simulink model "MVC2026_sim"  (R2023b)
settings: Solver=ode23t  StartTime=0.0  StopTime=inf  FixedStep=Ts  RelTol=1e-3
values from neighbouring files (symbols this model uses):
  saveDataSampling = 0.01    [main.m]
undefined symbols (not defined in the file or in its folder): BAT, BUS, CH, CTRLpmsm, DiscIntNeverNeededParam, EMS, LoadRef, MOT, TraceRef, Ts, VEH, WindRef
libraries: nesl_utility x50, fl_lib x28, ee_lib x19, simulink x9, slpidlib x5, eeTransforms x4, sdl_lib x4, batteryecm_lib x1, eeGeneralControl x1
(part 3 of 3)

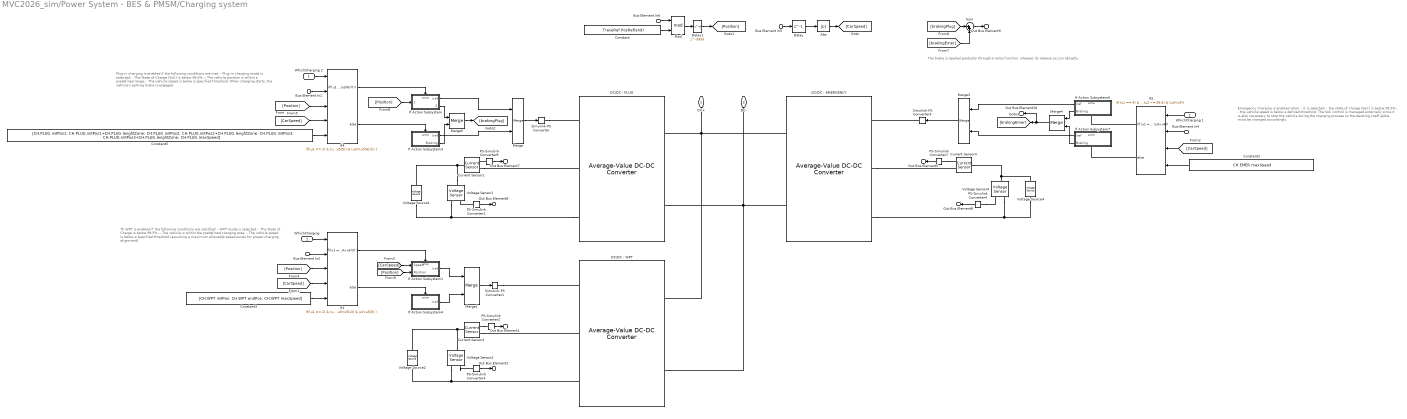
== system MVC2026_sim/Power System - BES & PMSM/Charging system ==
  note: Plug-in charging is enabled if the following conditions are met:
      | - Plug-in charging mode is selected;
      | - The State of Charge (SoC) is below 99.5%;
      | - The vehicle position is within a predefined range;
      | - The vehicle speed is below a specified threshold.
      |
      | When charging starts, the vehicle’s parking brake is engaged.
  note: Th WPT is enabled if the following conditions are satisfied:
      | - WPT mode is selected;
      | - The State of Charge is below 99.5%;
      | - The vehicle is within the predefined charging area;
      | - The vehicle speed is below a specified threshold (assuming a maximum
      |  allowable speed exists for proper charging alignment).
  note: Emergency charging is enabled when:
      | - it is selected;
      | - the state of charge (SoC) is below 99.5%;
      | - the vehicle speed is below a defined threshold.
      |
      | The SoC control is managed externally since it is also necessary
      | to stop the vehicle during the charging process so the derating coeff alpha
      | must be changed accordingly.
  note: The brake is applied gradually through a ramp function, whereas its release occurs abruptly.
  WhichCharging : Inport
  Bus Element In4 : Inport  Port=2  PortName=DAQ  Element=SoC_BP
  Bus Element In1 : Inport  Port=2  PortName=DAQ  Element=SoC_BP
  Bus Element In2 : Inport  Port=2  PortName=DAQ  Element=SoC_BP
  Bus Element In6 : Inport  Port=2  PortName=DAQ  Element=Position
  Bus Element In5 : Inport  Port=2  PortName=DAQ  Element=CarSpeed
  Abs : Abs  SaturateOnIntegerOverflow=off
  Constant : Constant  Value=TraceRef.PosRef(end)
  Constant2 : Constant  Value=CH.EMER.maxSpeed
  Constant3 : Constant  Value=[CH.WPT.initPos; CH.WPT.endPos; CH.WPT.maxSpeed]
  Constant5 : Constant  Value=[CH.PLUG.initPos1; CH.PLUG.initPos1+CH.PLUG.lenghtZone; CH.PLUG.initPos2; CH.PLUG.initPos2+CH.PLUG.lenghtZone; CH.PLUG.initPos3; CH.PLUG.initPos3+CH.PLUG.lenghtZone; CH.PLUG.maxSpeed]
  Current Sensor1 : fl_lib/Electrical/Electrical Sensors/Current Sensor
  Current Sensor2 : fl_lib/Electrical/Electrical Sensors/Current Sensor
  Current Sensor4 : fl_lib/Electrical/Electrical Sensors/Current Sensor
  DC/DC - EMERGENCY : ee_lib/Semiconductors & Converters/Converters/Average-Value DC-DC Converter  control_option=ee.enum.converters.controlinput.current  converter_type=ee.enum.converters.dcdctype.buck  efficiency_option=ee.enum.converters.efficiency.tabulated  efficiency_fixed=100  i_vec=CONV.EMER.I A  efficiency_vec=CONV.EMER.eta
      settings: InternalSimscapePortConfiguration="{\"Bottom\":[],\"Left\":[{\"id\":\"Iref\",\"label\":\"Iref\",\"type\":\"input\"},{\"id\":\"p1\",\"label\":\"1+\",\"type\":\"foundation.electrical.electrical\"},{\"id\":\"n1\",\"label\":\"1-\",\"type\":\"foundation.electrical.electrical\"}],\"Right\":[{\"id\":\"p2\",\"label\":\"2+\",\"type\":\"foundation.electrical.electrical\"},{\"id\":\"n2\",\"label\":\"2-\",\"type\":\"foundation.electrical.electrical\"}],\"Top\":[]}"
  DC/DC - PLUG : ee_lib/Semiconductors & Converters/Converters/Average-Value DC-DC Converter  control_option=ee.enum.converters.controlinput.current  converter_type=ee.enum.converters.dcdctype.buck  efficiency_option=ee.enum.converters.efficiency.tabulated  efficiency_fixed=100  i_vec=CONV.PLUG.I A  efficiency_vec=CONV.PLUG.eta
      settings: InternalSimscapePortConfiguration="{\"Bottom\":[],\"Left\":[{\"id\":\"Iref\",\"label\":\"Iref\",\"type\":\"input\"},{\"id\":\"p1\",\"label\":\"1+\",\"type\":\"foundation.electrical.electrical\"},{\"id\":\"n1\",\"label\":\"1-\",\"type\":\"foundation.electrical.electrical\"}],\"Right\":[{\"id\":\"p2\",\"label\":\"2+\",\"type\":\"foundation.electrical.electrical\"},{\"id\":\"n2\",\"label\":\"2-\",\"type\":\"foundation.electrical.electrical\"}],\"Top\":[]}"
  DC/DC - WPT : ee_lib/Semiconductors & Converters/Converters/Average-Value DC-DC Converter  control_option=ee.enum.converters.controlinput.current  converter_type=ee.enum.converters.dcdctype.buck  efficiency_option=ee.enum.converters.efficiency.tabulated  efficiency_fixed=100  i_vec=CONV.WPT.I A  efficiency_vec=CONV.WPT.eta
      settings: InternalSimscapePortConfiguration="{\"Bottom\":[],\"Left\":[{\"id\":\"Iref\",\"label\":\"Iref\",\"type\":\"input\"},{\"id\":\"p1\",\"label\":\"1+\",\"type\":\"foundation.electrical.electrical\"},{\"id\":\"n1\",\"label\":\"1-\",\"type\":\"foundation.electrical.electrical\"}],\"Right\":[{\"id\":\"p2\",\"label\":\"2+\",\"type\":\"foundation.electrical.electrical\"},{\"id\":\"n2\",\"label\":\"2-\",\"type\":\"foundation.electrical.electrical\"}],\"Top\":[]}"
  Delay : Delay  DelayLength=1  SampleTime=Ts
  Delay1 : Delay  DelayLength=3333  UseCircularBuffer=on  SampleTime=Ts
  If Action Subsystem : Subsystem  TreatAsAtomicUnit=on
  If Action Subsystem1 : Subsystem  TreatAsAtomicUnit=on
  If Action Subsystem3 : Subsystem  TreatAsAtomicUnit=on
  If Action Subsystem4 : Subsystem  TreatAsAtomicUnit=on
  If Action Subsystem6 : Subsystem  TreatAsAtomicUnit=on
  If Action Subsystem7 : Subsystem  TreatAsAtomicUnit=on
  If1 : If  NumInputs=5  IfExpression=(u1 == 2) & (u2 <= 99.5) & (u3>u5(1) & u3<u5(2)) & u4<u5(3)
  If3 : If  NumInputs=4  IfExpression=(u1 == 4) & (u2 <= 99.5) & (u3<u4)
  If4 : If  NumInputs=5  IfExpression=(u1 == 1) & (u2 <= 99.5) & (u4<u5(7)) & (((u3>u5(1)) & (u3<(u5(2)))) | ((u3>u5(3)) & (u3<(u5(4)))) | ((u3>u5(5)) & (u3<(u5(6)))))
  Merge{,1,3..5} (5 alike) : Merge
  Mod : Math  Operator=mod
  PS-Simulink Converter1 : nesl_utility/PS-Simulink Converter  PhysicalDomain=network_engine_domain  SubClassName=ps_output  LeftPortType=input  RightPortType=output  PseudoPeriodic=off  Frequencies=[]  VectorFormat=1-D array  Unit=V  AffineConversion=off
  PS-Simulink Converter2 : nesl_utility/PS-Simulink Converter  PhysicalDomain=network_engine_domain  SubClassName=ps_output  LeftPortType=input  RightPortType=output  PseudoPeriodic=off  Frequencies=[]  VectorFormat=1-D array  Unit=A  AffineConversion=off
  PS-Simulink Converter3 : nesl_utility/PS-Simulink Converter  PhysicalDomain=network_engine_domain  SubClassName=ps_output  LeftPortType=input  RightPortType=output  PseudoPeriodic=off  Frequencies=[]  VectorFormat=1-D array  Unit=V  AffineConversion=off
  PS-Simulink Converter4 : nesl_utility/PS-Simulink Converter  PhysicalDomain=network_engine_domain  SubClassName=ps_output  LeftPortType=input  RightPortType=output  PseudoPeriodic=off  Frequencies=[]  VectorFormat=1-D array  Unit=V  AffineConversion=off
  PS-Simulink Converter7 : nesl_utility/PS-Simulink Converter  PhysicalDomain=network_engine_domain  SubClassName=ps_output  LeftPortType=input  RightPortType=output  PseudoPeriodic=off  Frequencies=[]  VectorFormat=1-D array  Unit=A  AffineConversion=off
  PS-Simulink Converter9 : nesl_utility/PS-Simulink Converter  PhysicalDomain=network_engine_domain  SubClassName=ps_output  LeftPortType=input  RightPortType=output  PseudoPeriodic=off  Frequencies=[]  VectorFormat=1-D array  Unit=A  AffineConversion=off
  Simulink-PS Converter : nesl_utility/Simulink-PS Converter  PhysicalDomain=network_engine_domain  SubClassName=ps_input  LeftPortType=input  RightPortType=output  PseudoPeriodic=off  Frequencies=[]  NoiseDistribution=none  NoiseParameters=[]  Unit=A  AffineConversion=off  FilteringAndDerivatives=provide  SimscapeFilterOrder=1  InputFilterTimeConstant=0.001  UdotUserProvided=0
  Simulink-PS Converter1 : nesl_utility/Simulink-PS Converter  PhysicalDomain=network_engine_domain  SubClassName=ps_input  LeftPortType=input  RightPortType=output  PseudoPeriodic=off  Frequencies=[]  NoiseDistribution=none  NoiseParameters=[]  Unit=A  AffineConversion=off  FilteringAndDerivatives=provide  SimscapeFilterOrder=1  InputFilterTimeConstant=0.001  UdotUserProvided=0
  Simulink-PS Converter3 : nesl_utility/Simulink-PS Converter  PhysicalDomain=network_engine_domain  SubClassName=ps_input  LeftPortType=input  RightPortType=output  PseudoPeriodic=off  Frequencies=[]  NoiseDistribution=none  NoiseParameters=[]  Unit=A  AffineConversion=off  FilteringAndDerivatives=provide  SimscapeFilterOrder=1  InputFilterTimeConstant=0.001  UdotUserProvided=0
  Sum : Sum  Inputs=|++
  Voltage Sensor1 : fl_lib/Electrical/Electrical Sensors/Voltage Sensor
  Voltage Sensor2 : fl_lib/Electrical/Electrical Sensors/Voltage Sensor
  Voltage Sensor4 : fl_lib/Electrical/Electrical Sensors/Voltage Sensor
  Voltage Source1 : ee_lib/Sources/Voltage Source  dc_voltage=CH.PLUG.V V  ac_voltage=0 V  ac_shift=0 rad  ac_frequency=60 Hz  noise_mode=ee.enum.sources.noise.Disabled  PSD=0 V^2/Hz  sample_time=1e-3 s  repeatability=ee.enum.sources.repeatability.NotRepeatable  user_seed=0  auto_seed=545404223  i_specify=off  i_priority=None  i=0 A  i_nominal_specify=off  i_nominal_unit=A  i_nominal_value=1  v_specify=off  v_priority=None  v=0 V  v_nominal_specify=off  v_nominal_unit=V  v_nominal_value=1
  Voltage Source2 : ee_lib/Sources/Voltage Source  dc_voltage=CH.WPT.V V  ac_voltage=0 V  ac_shift=0 rad  ac_frequency=60 Hz  noise_mode=ee.enum.sources.noise.Disabled  PSD=0 V^2/Hz  sample_time=1e-3 s  repeatability=ee.enum.sources.repeatability.NotRepeatable  user_seed=0  auto_seed=3922919431  i_specify=off  i_priority=None  i=0 A  i_nominal_specify=off  i_nominal_unit=A  i_nominal_value=1  v_specify=off  v_priority=None  v=0 V  v_nominal_specify=off  v_nominal_unit=V  v_nominal_value=1
  Voltage Source4 : ee_lib/Sources/Voltage Source  dc_voltage=CH.EMER.V V  ac_voltage=0 V  ac_shift=0 rad  ac_frequency=60 Hz  noise_mode=ee.enum.sources.noise.Disabled  PSD=0 V^2/Hz  sample_time=1e-3 s  repeatability=ee.enum.sources.repeatability.NotRepeatable  user_seed=0  auto_seed=4144164703  i_specify=off  i_priority=None  i=0 A  i_nominal_specify=off  i_nominal_unit=A  i_nominal_value=1  v_specify=off  v_priority=None  v=0 V  v_nominal_specify=off  v_nominal_unit=V  v_nominal_value=1
  WhichCharging 1 : InportShadow
  WhichCharging 2 : InportShadow
  DC+ : PMIOPort  Side=Right
  DC- : PMIOPort  Port=2  Side=Right
  Out Bus Element7 : Outport  PortName=CH  Element=iPLUG
  Out Bus Element8 : Outport  PortName=CH  Element=vPLUG
  Out Bus Element1 : Outport  PortName=CH  Element=iWPT
  Out Bus Element2 : Outport  PortName=CH  Element=vWPT
  Out Bus Element5 : Outport  PortName=CH  Element=iEMERGENCY
  Out Bus Element6 : Outport  PortName=CH  Element=vEMERGENCY
  Out Bus Element9 : Outport  PortName=CH  Element=Braking
  Out Bus Element10 : Outport  PortName=CH  Element=EMERGENCYisON
  wires:
  WhichCharging 2/1 -> If4/1
  Bus Element In1/1 -> If4/2
  Bus Element In2/1 -> If1/2
  WhichCharging/1 -> If1/1
  If4/1 -> If Action Subsystem/Action
  If4/2 -> If Action Subsystem3/Action
  If Action Subsystem3/1(Iref) -> Merge/2
  If Action Subsystem/1(Iref) -> Merge/1
  If Action Subsystem1/1(Iref) -> Merge1/1
  If Action Subsystem4/1(Iref) -> Merge1/2
  If1/2 -> If Action Subsystem4/Action
  If1/1 -> If Action Subsystem1/Action
  Merge1/1 -> Simulink-PS Converter1/1
  Bus Element In6/1 -> Mod/1
  Constant/1 -> Mod/2
  Bus Element In5/1 -> Delay/1
  Delay/1 -> Abs/1
  Merge3/1 -> Simulink-PS Converter3/1
  If Action Subsystem/2(Braking) -> Merge5/1
  If Action Subsystem3/2(Braking) -> Merge5/2
  Constant5/1 -> If4/5
  If Action Subsystem7/2(Braking) -> Merge4/2
  If Action Subsystem6/2(Braking) -> Merge4/1
  If3/2 -> If Action Subsystem7/Action
  If Action Subsystem7/1(Iref) -> Merge3/2
  If Action Subsystem6/1(Iref) -> Merge3/1
  If3/1 -> If Action Subsystem6/Action
  Bus Element In4/1 -> If3/2
  Constant2/1 -> If3/4
  Merge4/1 -> Out Bus Element10/1, [brakingEmer]
  Constant3/1 -> If1/5
  Sum/1 -> Out Bus Element9/1
  Abs/1 -> [CarSpeed]
  [CarSpeed] -> If3/3
  [Position] -> If1/3
  [Position] -> If4/3
  Merge5/1 -> [brakingPlug]
  WhichCharging 1/1 -> If3/1
  [Position] -> If Action Subsystem/1(Position)
  [CarSpeed] -> If4/4
  [CarSpeed] -> If1/4
  [CarSpeed] -> If Action Subsystem1/1(Speed)
  Mod/1 -> Delay1/1
  Delay1/1 -> [Position]
  Merge/1 -> Simulink-PS Converter/1
  [brakingEmer] -> Sum/2
  [brakingPlug] -> Sum/1
  [Position] -> If Action Subsystem1/2(Position)
  PS-Simulink Converter9/1 -> Out Bus Element7/1
  PS-Simulink Converter1/1 -> Out Bus Element8/1
  PS-Simulink Converter2/1 -> Out Bus Element1/1
  PS-Simulink Converter3/1 -> Out Bus Element2/1
  PS-Simulink Converter4/1 -> Out Bus Element6/1
  PS-Simulink Converter7/1 -> Out Bus Element5/1
  connections:
  PS-Simulink Converter9/LConn1 -- Current Sensor1/RConn1
  Voltage Sensor1/LConn1 -- Voltage Source1/LConn1 -- Current Sensor1/LConn1
  PS-Simulink Converter1/LConn1 -- Voltage Sensor1/RConn1
  DC/DC - PLUG/LConn3 -- Voltage Source1/RConn1 -- Voltage Sensor1/RConn2
  Current Sensor1/RConn2 -- DC/DC - PLUG/LConn2
  Voltage Source2/LConn1 -- Voltage Sensor2/LConn1 -- Current Sensor2/LConn1
  Current Sensor2/RConn2 -- DC/DC - WPT/LConn2
  Voltage Sensor2/RConn1 -- PS-Simulink Converter3/LConn1
  Current Sensor2/RConn1 -- PS-Simulink Converter2/LConn1
  Voltage Source2/RConn1 -- Voltage Sensor2/RConn2 -- DC/DC - WPT/LConn3
  DC/DC - PLUG/RConn2 -- DC/DC - WPT/RConn2 -- DC/DC - EMERGENCY/RConn2 -- DC-/RConn1
  Simulink-PS Converter/RConn1 -- DC/DC - PLUG/LConn1
  Simulink-PS Converter1/RConn1 -- DC/DC - WPT/LConn1
  Simulink-PS Converter3/RConn1 -- DC/DC - EMERGENCY/LConn1
  Voltage Source4/LConn1 -- Current Sensor4/LConn1 -- Voltage Sensor4/LConn1
  Voltage Source4/RConn1 -- DC/DC - EMERGENCY/LConn3 -- Voltage Sensor4/RConn2
  PS-Simulink Converter4/LConn1 -- Voltage Sensor4/RConn1
  PS-Simulink Converter7/LConn1 -- Current Sensor4/RConn1
  DC/DC - EMERGENCY/LConn2 -- Current Sensor4/RConn2
  DC/DC - WPT/RConn1 -- DC/DC - PLUG/RConn1 -- DC/DC - EMERGENCY/RConn1 -- DC+/RConn1

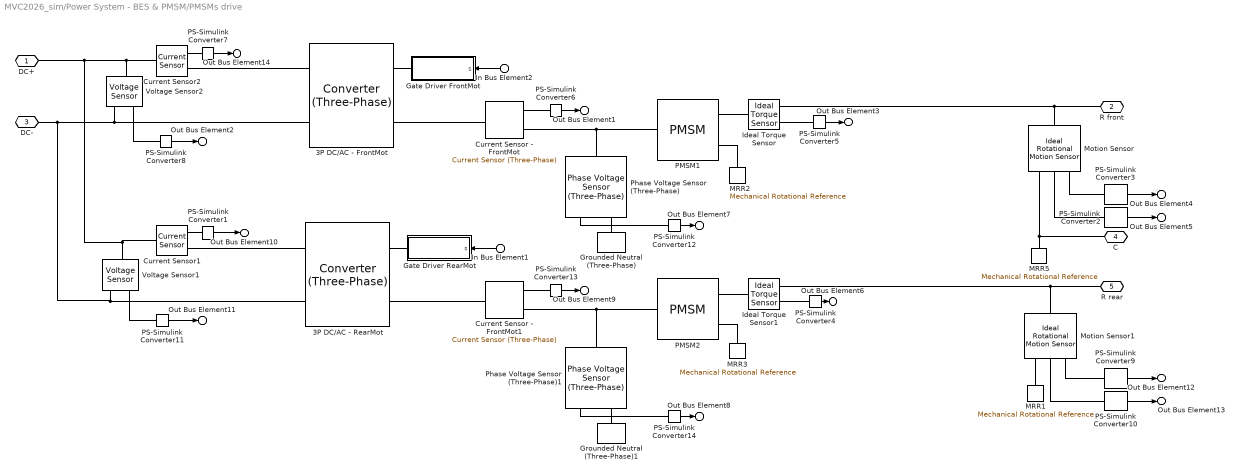
== system MVC2026_sim/Power System - BES & PMSM/PMSMs drive ==
  In Bus Element1 : Inport  PortName=CTRL  Element=swRearMot
  In Bus Element2 : Inport  PortName=CTRL  Element=swFrontMot
  3P DC/AC - FrontMot : ee_lib/Semiconductors & Converters/Converters/Converter (Three-Phase)  port_option=ee.enum.threePhasePort.composite  device_type=ee.enum.converters.switchingdevice.averaged  K=0  Vf=0.01 V  Ron=0.001 Ohm  Rds=0.001 Ohm  Goff=1e-6 1/Ohm  Vgt=1 V  Vgt_off=-1 V  Ih=1 A  Vth=0.5 V  diode_param=ee.enum.converters.protectiondiode.none  diode_Vf=0.8 V  diode_Ron=0.001 Ohm  diode_Goff=1e-5 1/Ohm  diode_C=50 nF  diode_iRM=-235 A  diode_iF=300 A  diode_idot=-50 A/us  diode_trr_param=ee.enum.converters.diodetrr.trr_factor  diode_trr_factor=3  diode_trr=15 us  diode_Qrr=1500 s*uA  snubber_type=ee.enum.converters.snubber.exclude  Cs=1e-7 F  Rs=0.1 Ohm
  3P DC/AC - RearMot : ee_lib/Semiconductors & Converters/Converters/Converter (Three-Phase)  port_option=ee.enum.threePhasePort.composite  device_type=ee.enum.converters.switchingdevice.averaged  K=0  Vf=0.01 V  Ron=0.001 Ohm  Rds=0.001 Ohm  Goff=1e-6 1/Ohm  Vgt=1 V  Vgt_off=-1 V  Ih=1 A  Vth=0.5 V  diode_param=ee.enum.converters.protectiondiode.none  diode_Vf=0.01 V  diode_Ron=0.001 Ohm  diode_Goff=1e-5 1/Ohm  diode_C=50 nF  diode_iRM=-235 A  diode_iF=300 A  diode_idot=-50 A/us  diode_trr_param=ee.enum.converters.diodetrr.trr_factor  diode_trr_factor=3  diode_trr=15 us  diode_Qrr=1500 s*uA  snubber_type=ee.enum.converters.snubber.exclude  Cs=1e-7 F  Rs=0.1 Ohm
  Current Sensor - FrontMot : ee_lib/Sensors & Transducers/Current Sensor (Three-Phase)
  Current Sensor - FrontMot1 : ee_lib/Sensors & Transducers/Current Sensor (Three-Phase)
  Current Sensor1 : fl_lib/Electrical/Electrical Sensors/Current Sensor
  Current Sensor2 : fl_lib/Electrical/Electrical Sensors/Current Sensor
  Gate Driver FrontMot : Subsystem
  Gate Driver RearMot : Subsystem
  Grounded Neutral (Three-Phase) : ee_lib/Connectors & References/Grounded Neutral (Three-Phase)
  Grounded Neutral (Three-Phase)1 : ee_lib/Connectors & References/Grounded Neutral (Three-Phase)
  Ideal Torque Sensor : fl_lib/Mechanical/Mechanical Sensors/Ideal Torque Sensor
  Ideal Torque Sensor1 : fl_lib/Mechanical/Mechanical Sensors/Ideal Torque Sensor
  MRR{1..3,5} (4 alike) : fl_lib/Mechanical/Rotational Elements/Mechanical Rotational Reference
  Motion Sensor : fl_lib/Mechanical/Mechanical Sensors/Ideal Rotational Motion Sensor  reference=foundation.enum.MeasurementReference.difference  acceleration_port=false  velocity_port=true  position_port=true  wrap_angle=simscape.enum.onoff.off  offset=0 rad
  Motion Sensor1 : fl_lib/Mechanical/Mechanical Sensors/Ideal Rotational Motion Sensor  reference=foundation.enum.MeasurementReference.difference  acceleration_port=false  velocity_port=true  position_port=true  wrap_angle=simscape.enum.onoff.off  offset=0 rad
  PMSM1 : ee_lib/Electromechanical/Permanent Magnet/PMSM  port_option=ee.enum.threePhasePort.composite  winding_type=ee.enum.statorconnection.wye  machine_param=ee.enum.pmsm.parameterization.constant  nPolePairs=MOT.Front.p  pmflux_param=ee.enum.pmflux.fluxlinkage  pm_flux_linkage=MOT.Front.PMflux Wb  torque_constant=0.18 N*m/A  back_emf_constant=0.18 V*s/rad  stator_param=ee.enum.statorparam.LdLqL0  Ld=MOT.Front.Ld H  Lq=MOT.Front.Lq H  idVec=[-200, 0, 200] A  iqVec=[-200, 0, 200] A  LdMatrix=0.0002 * ones(3, 3) H  LqMatrix=0.0002 * ones(3, 3) H  PmMatrix=0.1 * ones(3, 3) Wb  ktMatrix=0.18 * ones(3, 3) N*m/A  keMatrix=0.18 * ones(3, 3) V*s/rad  L0=MOT.L0 H  Ls=0.0002 H  Lm=-0.00002 H  Ms=0.00002 H  Rs=MOT.Front.R Ohm  zero_sequence=ee.enum.park.zerosequence.exclude  axes_param=ee.enum.rotorangle.daxis  loss_param=ee.enum.ironloss.empirical  losses_oc=[MOT.Front.P_hyst_OC, MOT.Front.P_eddy_OC, MOT.Front.P_exce_OC] W  losses_sc=[MOT.Front.P_hyst_SC, MOT.Front.P_eddy_SC, MOT.Front.P_exce_SC] W  f_losses=60 Hz  Isc_losses=95 A  J=MOT.Front.J kg*m^2  lam=MOT.Front.D N*m*s/rad  i_d_specify=off  i_d_priority=None  i_d=0 A  i_d_nominal_specify=off  i_d_nominal_unit=A  i_d_nominal_value=1  i_q_specify=off  i_q_priority=None  i_q=0 A  i_q_nominal_specify=off  i_q_nominal_unit=A  i_q_nominal_value=1  torque_specify=off  torque_priority=None  torque=0 N*m  torque_nominal_specify=off  torque_nominal_unit=N*m  torque_nominal_value=1  angular_velocity_specify=off  angular_velocity_priority=High  angular_velocity=0 rpm  angular_velocity_nominal_specify=off  angular_velocity_nominal_unit=rpm  angular_velocity_nominal_value=1  angular_position_specify=off  angular_position_priority=High  angular_position=0 deg  angular_position_nominal_specify=off  angular_position_nominal_unit=deg  angular_position_nominal_value=1  alpha=3.93e-3 1/K  alpha_flux=-0.001 1/K  Tmeas=298.15 K  stator_thermal_mass=100 J/K  rotor_thermal_mass=200 J/K  Rm_percent_rotor=90  Rd_percent_rotor=30  temperatureA_specify=off  temperatureA_priority=High  temperatureA=25 degC  temperatureA_nominal_specify=off  temperatureA_nominal_unit=degC  temperatureA_nominal_value=1  temperatureB_specify=off  temperatureB_priority=High  temperatureB=25 degC  temperatureB_nominal_specify=off  temperatureB_nominal_unit=degC  temperatureB_nominal_value=1  temperatureC_specify=off  temperatureC_priority=High  temperatureC=25 degC  temperatureC_nominal_specify=off  temperatureC_nominal_unit=degC  temperatureC_nominal_value=1  temperatureR_specify=off  temperatureR_priority=High  temperatureR=25 degC  temperatureR_nominal_specify=off  temperatureR_nominal_unit=degC  temperatureR_nominal_value=1
      settings: InternalSimscapePortConfiguration="{\"Bottom\":[],\"Left\":[{\"id\":\"N\",\"label\":\"~\",\"type\":\"foundation.electrical.three_phase\"}],\"Right\":[{\"id\":\"R\",\"label\":\"R\",\"type\":\"foundation.mechanical.rotational.rotational\"},{\"id\":\"C\",\"label\":\"C\",\"type\":\"foundation.mechanical.rotational.rotational\"}],\"Top\":[]}"
  PMSM2 : ee_lib/Electromechanical/Permanent Magnet/PMSM  port_option=ee.enum.threePhasePort.composite  winding_type=ee.enum.statorconnection.wye  machine_param=ee.enum.pmsm.parameterization.constant  nPolePairs=MOT.Rear.p  pmflux_param=ee.enum.pmflux.fluxlinkage  pm_flux_linkage=MOT.Rear.PMflux Wb  torque_constant=0.18 N*m/A  back_emf_constant=0.18 V*s/rad  stator_param=ee.enum.statorparam.LdLqL0  Ld=MOT.Rear.Ld H  Lq=MOT.Rear.Lq H  idVec=[-200, 0, 200] A  iqVec=[-200, 0, 200] A  LdMatrix=0.0002 * ones(3, 3) H  LqMatrix=0.0002 * ones(3, 3) H  PmMatrix=0.1 * ones(3, 3) Wb  ktMatrix=0.18 * ones(3, 3) N*m/A  keMatrix=0.18 * ones(3, 3) V*s/rad  L0=MOT.L0 H  Ls=0.0002 H  Lm=-0.00002 H  Ms=0.00002 H  Rs=MOT.Rear.R Ohm  zero_sequence=ee.enum.park.zerosequence.exclude  axes_param=ee.enum.rotorangle.daxis  loss_param=ee.enum.ironloss.empirical  losses_oc=[MOT.Rear.P_hyst_OC, MOT.Rear.P_eddy_OC, MOT.Rear.P_exce_OC] W  losses_sc=[MOT.Rear.P_hyst_SC, MOT.Rear.P_eddy_SC, MOT.Rear.P_exce_SC] W  f_losses=60 Hz  Isc_losses=95 A  J=MOT.Rear.J kg*m^2  lam=MOT.Rear.D N*m*s/rad  i_d_specify=off  i_d_priority=None  i_d=0 A  i_d_nominal_specify=off  i_d_nominal_unit=A  i_d_nominal_value=1  i_q_specify=off  i_q_priority=None  i_q=0 A  i_q_nominal_specify=off  i_q_nominal_unit=A  i_q_nominal_value=1  torque_specify=off  torque_priority=None  torque=0 N*m  torque_nominal_specify=off  torque_nominal_unit=N*m  torque_nominal_value=1  angular_velocity_specify=off  angular_velocity_priority=High  angular_velocity=0 rpm  angular_velocity_nominal_specify=off  angular_velocity_nominal_unit=rpm  angular_velocity_nominal_value=1  angular_position_specify=off  angular_position_priority=High  angular_position=0 deg  angular_position_nominal_specify=off  angular_position_nominal_unit=deg  angular_position_nominal_value=1  alpha=3.93e-3 1/K  alpha_flux=-0.001 1/K  Tmeas=298.15 K  stator_thermal_mass=100 J/K  rotor_thermal_mass=200 J/K  Rm_percent_rotor=90  Rd_percent_rotor=30  temperatureA_specify=off  temperatureA_priority=High  temperatureA=25 degC  temperatureA_nominal_specify=off  temperatureA_nominal_unit=degC  temperatureA_nominal_value=1  temperatureB_specify=off  temperatureB_priority=High  temperatureB=25 degC  temperatureB_nominal_specify=off  temperatureB_nominal_unit=degC  temperatureB_nominal_value=1  temperatureC_specify=off  temperatureC_priority=High  temperatureC=25 degC  temperatureC_nominal_specify=off  temperatureC_nominal_unit=degC  temperatureC_nominal_value=1  temperatureR_specify=off  temperatureR_priority=High  temperatureR=25 degC  temperatureR_nominal_specify=off  temperatureR_nominal_unit=degC  temperatureR_nominal_value=1
      settings: InternalSimscapePortConfiguration="{\"Bottom\":[],\"Left\":[{\"id\":\"N\",\"label\":\"~\",\"type\":\"foundation.electrical.three_phase\"}],\"Right\":[{\"id\":\"R\",\"label\":\"R\",\"type\":\"foundation.mechanical.rotational.rotational\"},{\"id\":\"C\",\"label\":\"C\",\"type\":\"foundation.mechanical.rotational.rotational\"}],\"Top\":[]}"
  PS-Simulink Converter{1,6..7,13} (4 alike) : nesl_utility/PS-Simulink Converter  PhysicalDomain=network_engine_domain  SubClassName=ps_output  LeftPortType=input  RightPortType=output  PseudoPeriodic=off  Frequencies=[]  VectorFormat=1-D array  Unit=A  AffineConversion=off
  PS-Simulink Converter10 : nesl_utility/PS-Simulink Converter  PhysicalDomain=network_engine_domain  SubClassName=ps_output  LeftPortType=input  RightPortType=output  PseudoPeriodic=off  Frequencies=[]  VectorFormat=1-D array  Unit=rad/s  AffineConversion=off
  PS-Simulink Converter{8,11..12,14} (4 alike) : nesl_utility/PS-Simulink Converter  PhysicalDomain=network_engine_domain  SubClassName=ps_output  LeftPortType=input  RightPortType=output  PseudoPeriodic=off  Frequencies=[]  VectorFormat=1-D array  Unit=V  AffineConversion=off
  PS-Simulink Converter2 : nesl_utility/PS-Simulink Converter  PhysicalDomain=network_engine_domain  SubClassName=ps_output  LeftPortType=input  RightPortType=output  PseudoPeriodic=off  Frequencies=[]  VectorFormat=1-D array  Unit=rad/s  AffineConversion=off
  PS-Simulink Converter3 : nesl_utility/PS-Simulink Converter  PhysicalDomain=network_engine_domain  SubClassName=ps_output  LeftPortType=input  RightPortType=output  PseudoPeriodic=off  Frequencies=[]  VectorFormat=1-D array  Unit=rad  AffineConversion=off
  PS-Simulink Converter4 : nesl_utility/PS-Simulink Converter  PhysicalDomain=network_engine_domain  SubClassName=ps_output  LeftPortType=input  RightPortType=output  PseudoPeriodic=off  Frequencies=[]  VectorFormat=1-D array  Unit=N*m  AffineConversion=off
  PS-Simulink Converter5 : nesl_utility/PS-Simulink Converter  PhysicalDomain=network_engine_domain  SubClassName=ps_output  LeftPortType=input  RightPortType=output  PseudoPeriodic=off  Frequencies=[]  VectorFormat=1-D array  Unit=N*m  AffineConversion=off
  PS-Simulink Converter9 : nesl_utility/PS-Simulink Converter  PhysicalDomain=network_engine_domain  SubClassName=ps_output  LeftPortType=input  RightPortType=output  PseudoPeriodic=off  Frequencies=[]  VectorFormat=1-D array  Unit=rad  AffineConversion=off
  Phase Voltage Sensor (Three-Phase) : ee_lib/Sensors & Transducers/Phase Voltage Sensor (Three-Phase)
  Phase Voltage Sensor (Three-Phase)1 : ee_lib/Sensors & Transducers/Phase Voltage Sensor (Three-Phase)
  Voltage Sensor1 : fl_lib/Electrical/Electrical Sensors/Voltage Sensor
  Voltage Sensor2 : fl_lib/Electrical/Electrical Sensors/Voltage Sensor
  DC+ : PMIOPort  Side=Left
  R front : PMIOPort  Port=2  Side=Right
  DC- : PMIOPort  Port=3  Side=Left
  C : PMIOPort  Port=4  Side=Right
  R rear : PMIOPort  Port=5  Side=Right
  Out Bus Element14 : Outport  PortName=DC  Element=iFrontMot
  Out Bus Element10 : Outport  PortName=DC  Element=iRearMot
  Out Bus Element11 : Outport  PortName=DC  Element=vRearMot
  Out Bus Element2 : Outport  PortName=DC  Element=vFrontMot
  Out Bus Element1 : Outport  Port=2  PortName=PMSM  Element=iFrontMot
  Out Bus Element9 : Outport  Port=2  PortName=PMSM  Element=iRearMot
  Out Bus Element3 : Outport  Port=2  PortName=PMSM  Element=TeFrontMot
  Out Bus Element4 : Outport  Port=2  PortName=PMSM  Element=thmFrontMot
  Out Bus Element5 : Outport  Port=2  PortName=PMSM  Element=wmFrontMot
  Out Bus Element6 : Outport  Port=2  PortName=PMSM  Element=TeRearMot
  Out Bus Element7 : Outport  Port=2  PortName=PMSM  Element=vFrontMot
  Out Bus Element8 : Outport  Port=2  PortName=PMSM  Element=vRearMot
  Out Bus Element12 : Outport  Port=2  PortName=PMSM  Element=thmRearMot
  Out Bus Element13 : Outport  Port=2  PortName=PMSM  Element=wmRearMot
  wires:
  PS-Simulink Converter11/1 -> Out Bus Element11/1
  PS-Simulink Converter13/1 -> Out Bus Element9/1
  PS-Simulink Converter7/1 -> Out Bus Element14/1
  PS-Simulink Converter8/1 -> Out Bus Element2/1
  In Bus Element1/1 -> Gate Driver RearMot/1(s)
  PS-Simulink Converter1/1 -> Out Bus Element10/1
  In Bus Element2/1 -> Gate Driver FrontMot/1(s)
  PS-Simulink Converter2/1 -> Out Bus Element5/1
  PS-Simulink Converter3/1 -> Out Bus Element4/1
  PS-Simulink Converter12/1 -> Out Bus Element7/1
  PS-Simulink Converter14/1 -> Out Bus Element8/1
  PS-Simulink Converter4/1 -> Out Bus Element6/1
  PS-Simulink Converter9/1 -> Out Bus Element12/1
  PS-Simulink Converter10/1 -> Out Bus Element13/1
  PS-Simulink Converter5/1 -> Out Bus Element3/1
  PS-Simulink Converter6/1 -> Out Bus Element1/1
  connections:
  Current Sensor - FrontMot1/RConn1 -- PS-Simulink Converter13/LConn1
  3P DC/AC - FrontMot/LConn2 -- Current Sensor - FrontMot/LConn1
  Current Sensor2/RConn2 -- 3P DC/AC - FrontMot/RConn1
  Current Sensor2/LConn1 -- Voltage Sensor1/LConn1 -- Current Sensor1/LConn1 -- DC+/RConn1 -- Voltage Sensor2/LConn1
  Current Sensor1/RConn1 -- PS-Simulink Converter1/LConn1
  PS-Simulink Converter6/LConn1 -- Current Sensor - FrontMot/RConn1
  3P DC/AC - FrontMot/LConn1 -- Gate Driver FrontMot/RConn1
  Voltage Sensor2/RConn2 -- Voltage Sensor1/RConn2 -- 3P DC/AC - RearMot/RConn2 -- DC-/RConn1 -- 3P DC/AC - FrontMot/RConn2
  3P DC/AC - RearMot/LConn1 -- Gate Driver RearMot/RConn1
  PS-Simulink Converter7/LConn1 -- Current Sensor2/RConn1
  Voltage Sensor1/RConn1 -- PS-Simulink Converter11/LConn1
  Current Sensor - FrontMot1/LConn1 -- 3P DC/AC - RearMot/LConn2
  Current Sensor1/RConn2 -- 3P DC/AC - RearMot/RConn1
  Phase Voltage Sensor (Three-Phase)/LConn1 -- PMSM1/LConn1 -- Current Sensor - FrontMot/RConn2
  PMSM2/LConn1 -- Current Sensor - FrontMot1/RConn2 -- Phase Voltage Sensor (Three-Phase)1/LConn1
  PS-Simulink Converter8/LConn1 -- Voltage Sensor2/RConn1
  PS-Simulink Converter3/LConn1 -- Motion Sensor/RConn3
  PS-Simulink Converter5/LConn1 -- Ideal Torque Sensor/RConn2
  PS-Simulink Converter2/LConn1 -- Motion Sensor/RConn2
  PMSM1/RConn1 -- Ideal Torque Sensor/LConn1
  MRR2/LConn1 -- PMSM1/RConn2
  MRR3/LConn1 -- PMSM2/RConn2
  Ideal Torque Sensor1/RConn2 -- PS-Simulink Converter4/LConn1
  Ideal Torque Sensor1/LConn1 -- PMSM2/RConn1
  Grounded Neutral (Three-Phase)/LConn1 -- Phase Voltage Sensor (Three-Phase)/RConn2
  PS-Simulink Converter12/LConn1 -- Phase Voltage Sensor (Three-Phase)/RConn1
  PS-Simulink Converter14/LConn1 -- Phase Voltage Sensor (Three-Phase)1/RConn1
  Grounded Neutral (Three-Phase)1/LConn1 -- Phase Voltage Sensor (Three-Phase)1/RConn2
  Motion Sensor/RConn1 -- MRR5/LConn1 -- C/RConn1
  Motion Sensor1/RConn1 -- MRR1/LConn1
  R rear/RConn1 -- Motion Sensor1/LConn1 -- Ideal Torque Sensor1/RConn1
  R front/RConn1 -- Ideal Torque Sensor/RConn1 -- Motion Sensor/LConn1
  Motion Sensor1/RConn2 -- PS-Simulink Converter10/LConn1
  Motion Sensor1/RConn3 -- PS-Simulink Converter9/LConn1

== system MVC2026_sim/Profile generation/If Action Subsystem6 ==
  Action Port : ActionPort  ActionPortLabel=if((u1<u3(1) & u2==0) | (u2==1 & (u1<u3(2))))
  Constant1 : Constant
  Constant2 : Constant  Value=4
  Emer_active : Outport
  WhichCharging_ : Outport  Port=2
  wires:
  Constant1/1 -> Emer_active/1
  Constant2/1 -> WhichCharging_/1

== system MVC2026_sim/Profile generation/If Action Subsystem7 ==
  WhichCharging : Inport
  Action Port : ActionPort  ActionPortLabel=else
  Constant1 : Constant  Value=0
  Emer_active : Outport
  WhichCharging_ : Outport  Port=2
  wires:
  Constant1/1 -> Emer_active/1
  WhichCharging/1 -> WhichCharging_/1

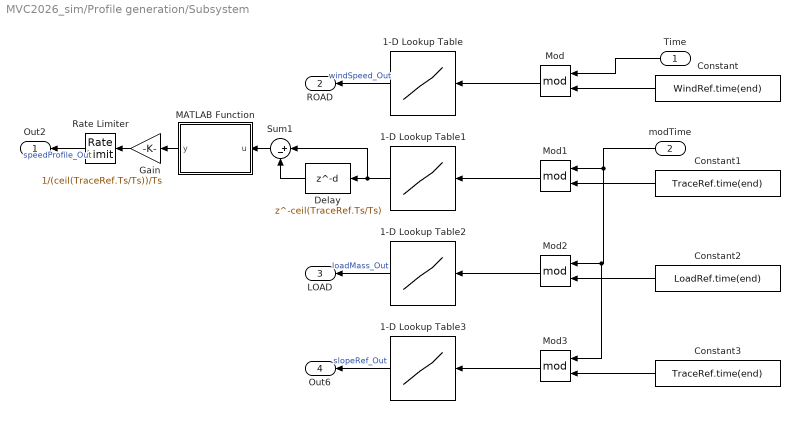
== system MVC2026_sim/Profile generation/Subsystem ==
  Time : Inport
  modTime : Inport  Port=2
  1-D Lookup Table : Lookup_n-D  NumberOfTableDimensions=1  BreakpointsForDimension1=WindRef.time  BeginIndexSearchUsingPreviousIndexResult=on  Table=WindRef.values  InterpMethod=Linear Lagrange  InternalRulePriority=Speed  RndMeth=Simplest
  1-D Lookup Table1 : Lookup_n-D  NumberOfTableDimensions=1  BreakpointsForDimension1=TraceRef.time  BeginIndexSearchUsingPreviousIndexResult=on  Table=TraceRef.PosRef  InterpMethod=Linear Lagrange  InternalRulePriority=Speed  RndMeth=Simplest
  1-D Lookup Table2 : Lookup_n-D  NumberOfTableDimensions=1  BreakpointsForDimension1=LoadRef.time  BeginIndexSearchUsingPreviousIndexResult=on  Table=LoadRef.values  InterpMethod=Linear Lagrange  InternalRulePriority=Speed  RndMeth=Simplest
  1-D Lookup Table3 : Lookup_n-D  NumberOfTableDimensions=1  BreakpointsForDimension1=TraceRef.time  BeginIndexSearchUsingPreviousIndexResult=on  Table=TraceRef.SlopeRef  InterpMethod=Linear Lagrange  InternalRulePriority=Speed  RndMeth=Simplest
  Constant : Constant  Value=WindRef.time(end)
  Constant1 : Constant  Value=TraceRef.time(end)
  Constant2 : Constant  Value=LoadRef.time(end)
  Constant3 : Constant  Value=TraceRef.time(end)
  Delay : Delay  DelayLength=ceil(TraceRef.Ts/Ts)  UseCircularBuffer=on
  Gain : Gain  Gain=1/(ceil(TraceRef.Ts/Ts))/Ts
  MATLAB Function : MATLAB Function  TreatAsAtomicUnit=on
  Mod{,1..3} (4 alike) : Math  Operator=mod
  Rate Limiter : RateLimiter  RisingSlewLimit=1000  FallingSlewLimit=-1000  SampleTimeMode=inherited
  Sum1 : Sum  Inputs=|+-
  Out2 : Outport
  ROAD : Outport  Port=2
  LOAD : Outport  Port=3
  Out6 : Outport  Port=4
  wires:
  Constant/1 -> Mod/2
  Constant2/1 -> Mod2/2
  Constant1/1 -> Mod1/2
  modTime/1 -> Mod3/1, Mod2/1, Mod1/1
  Rate Limiter/1 -> Out2/1  "speedProfile_Out"
  Time/1 -> Mod/1
  1-D Lookup Table3/1 -> Out6/1  "slopeRef_Out"
  1-D Lookup Table2/1 -> LOAD/1  "loadMass_Out"
  Constant3/1 -> Mod3/2
  1-D Lookup Table/1 -> ROAD/1  "windSpeed_Out"
  Mod/1 -> 1-D Lookup Table/1
  Mod1/1 -> 1-D Lookup Table1/1
  Mod2/1 -> 1-D Lookup Table2/1
  Mod3/1 -> 1-D Lookup Table3/1
  Gain/1 -> Rate Limiter/1
  1-D Lookup Table1/1 -> Delay/1, Sum1/1
  Delay/1 -> Sum1/2
  MATLAB Function/1(y) -> Gain/1
  Sum1/1 -> MATLAB Function/1(u)

== system MVC2026_sim/Power System - BES & PMSM/Charging system/If Action Subsystem ==
  note: If the system is in this block, it means the vehicle is in a condition
      | to recharge via the plug. However, it is necessary to distinguish
      | whether the plug is a fast or a slow one.
      | Since there is only one fast charging station, the system checks
      | whether it is within the range of the fast charger.
      | If not, it sets the charging current to the value corresponding to
      | slow charging.
  Position : Inport
  Action Port : ActionPort  ActionPortLabel=|
      | if((u1 == 1) & (u2 <= 99.5) & (u4<u5(7)) & (((u3>u5(1)) & (u3<(u5(2)))) | ((u3>u5(3)) & (u3<(u5(4)))) | ((u3>u5(5)) & (u3<(u5(6)))))
      | )
  Constant1 : Constant  SampleTime=-1
  Constant2 : Constant  Value=[CH.PLUG.initPos1; CH.PLUG.initPos1+CH.PLUG.lenghtZone;]
  If : If  NumInputs=2  IfExpression=(u1 > u2(1)) & (u1 < (u2(2)))
  If Action Subsystem : Subsystem  TreatAsAtomicUnit=on
  If Action Subsystem3 : Subsystem  TreatAsAtomicUnit=on
  Merge : Merge
  Rate Limiter : RateLimiter  RisingSlewLimit=0.3  FallingSlewLimit=-0.3  SampleTimeMode=inherited
  Iref : Outport
  Braking : Outport  Port=2
  wires:
  Constant1/1 -> Rate Limiter/1
  Rate Limiter/1 -> Braking/1
  Position/1 -> If/1
  Constant2/1 -> If/2
  If/1 -> If Action Subsystem/Action
  If Action Subsystem/1(Iref) -> Merge/1
  If Action Subsystem3/1(Iref) -> Merge/2
  If/2 -> If Action Subsystem3/Action
  Merge/1 -> Iref/1

== system MVC2026_sim/Power System - BES & PMSM/Charging system/If Action Subsystem1 ==
  note: I modeled the charging current (i.e., the power) as a function of the vehicle
      | speed, with maximum current delivered at zero speed and zero current at the
      | maximum allowable speed.
      | In addition, the current is modulated based on the vehicle's position following
      | a predefined spatial profile implemented in MATLAB.
  Speed : Inport
  Position : Inport  Port=2
  Action Port : ActionPort  ActionPortLabel=if((u1 == 2) & (u2 <= 99.5) & (u3>u5(1) & u3<u5(2)) & u4<u5(3) )
  1-D Lookup Table : Lookup_n-D  NumberOfTableDimensions=1  BreakpointsForDimension1=CH.WPT.CHprof.th  Table=CH.WPT.CHprof.gain  InternalRulePriority=Speed  RndMeth=Simplest
  Constant : Constant  Value=CH.WPT.I
  Constant1 : Constant  Value=CH.WPT.maxSpeed
  Constant2 : Constant  Value=CH.WPT.initPos
  Constant3 : Constant  Value=CH.WPT.CHprof.th(end)
  Gain : Gain  Gain=1/(CH.WPT.maxSpeed)
  Mod : Math  Operator=mod
  Product : Product
  Product1 : Product
  Saturation : Saturate  UpperLimit=Inf  LowerLimit=0
  Saturation1 : Saturate  UpperLimit=Inf  LowerLimit=0
  Sum : Sum  Inputs=-+|
  Sum1 : Sum  Inputs=|+-
  Iref : Outport
  wires:
  Constant/1 -> Product/1
  Constant1/1 -> Sum/2
  Speed/1 -> Saturation1/1
  Sum/1 -> Saturation/1
  Saturation1/1 -> Sum/1
  Saturation/1 -> Gain/1
  Gain/1 -> Product/2
  Product/1 -> Product1/1
  Position/1 -> Sum1/1
  Constant2/1 -> Sum1/2
  Sum1/1 -> Mod/1
  Constant3/1 -> Mod/2
  Mod/1 -> 1-D Lookup Table/1
  Product1/1 -> Iref/1
  1-D Lookup Table/1 -> Product1/2

== system MVC2026_sim/Power System - BES & PMSM/Charging system/If Action Subsystem3 ==
  Action Port : ActionPort  ActionPortLabel=else
  Constant : Constant  Value=0
  Constant1 : Constant  Value=0
  Iref : Outport
  Braking : Outport  Port=2
  wires:
  Constant/1 -> Iref/1
  Constant1/1 -> Braking/1

== system MVC2026_sim/Power System - BES & PMSM/Charging system/If Action Subsystem4 ==
  Action Port : ActionPort  ActionPortLabel=else
  Constant : Constant  Value=0
  Iref : Outport
  wires:
  Constant/1 -> Iref/1

== system MVC2026_sim/Power System - BES & PMSM/Charging system/If Action Subsystem6 ==
  Action Port : ActionPort  ActionPortLabel=if((u1 == 4) & (u2 <= 99.5) & (u3<u4))
  Constant : Constant  Value=CH.EMER.I
  Constant1 : Constant
  Rate Limiter : RateLimiter  RisingSlewLimit=0.3  FallingSlewLimit=-0.3  SampleTimeMode=inherited
  Rate Limiter1 : RateLimiter  RisingSlewLimit=10  FallingSlewLimit=-10  SampleTimeMode=inherited
  Iref : Outport
  Braking : Outport  Port=2
  wires:
  Constant/1 -> Rate Limiter1/1
  Constant1/1 -> Rate Limiter/1
  Rate Limiter/1 -> Braking/1
  Rate Limiter1/1 -> Iref/1

== system MVC2026_sim/Power System - BES & PMSM/Charging system/If Action Subsystem7 ==
  Action Port : ActionPort  ActionPortLabel=else
  Constant : Constant  Value=0
  Constant1 : Constant  Value=0
  Iref : Outport
  Braking : Outport  Port=2
  wires:
  Constant/1 -> Iref/1
  Constant1/1 -> Braking/1

== system MVC2026_sim/Power System - BES & PMSM/PMSMs drive/Gate Driver FrontMot ==
  s : Inport
  Demux : Demux  Outputs=6
  Simulink-PS Converter{1..6} (6 alike) : nesl_utility/Simulink-PS Converter  PhysicalDomain=network_engine_domain  SubClassName=ps_input  LeftPortType=input  RightPortType=output  PseudoPeriodic=off  Frequencies=[]  NoiseDistribution=none  NoiseParameters=[]  Unit=1  AffineConversion=off  FilteringAndDerivatives=zero  SimscapeFilterOrder=1  InputFilterTimeConstant=0.001  UdotUserProvided=1
  Six-Pulse Gate Multiplexer : ee_lib/Semiconductors & Converters/Converters/Six-Pulse Gate Multiplexer  port_option=ee.enum.controlport.ps
  g : PMIOPort  Side=Right
  wires:
  s/1 -> Demux/1
  Demux/1 -> Simulink-PS Converter1/1
  Demux/2 -> Simulink-PS Converter2/1
  Demux/5 -> Simulink-PS Converter5/1
  Demux/6 -> Simulink-PS Converter6/1
  Demux/3 -> Simulink-PS Converter3/1
  Demux/4 -> Simulink-PS Converter4/1
  connections:
  Six-Pulse Gate Multiplexer/LConn5 -- Simulink-PS Converter5/RConn1
  Six-Pulse Gate Multiplexer/LConn2 -- Simulink-PS Converter2/RConn1
  Simulink-PS Converter6/RConn1 -- Six-Pulse Gate Multiplexer/LConn6
  Six-Pulse Gate Multiplexer/RConn1 -- g/RConn1
  Six-Pulse Gate Multiplexer/LConn3 -- Simulink-PS Converter3/RConn1
  Six-Pulse Gate Multiplexer/LConn1 -- Simulink-PS Converter1/RConn1
  Six-Pulse Gate Multiplexer/LConn4 -- Simulink-PS Converter4/RConn1

== system MVC2026_sim/Power System - BES & PMSM/PMSMs drive/Gate Driver RearMot ==
  s : Inport
  Demux : Demux  Outputs=6
  Simulink-PS Converter{1..6} (6 alike) : nesl_utility/Simulink-PS Converter  PhysicalDomain=network_engine_domain  SubClassName=ps_input  LeftPortType=input  RightPortType=output  PseudoPeriodic=off  Frequencies=[]  NoiseDistribution=none  NoiseParameters=[]  Unit=1  AffineConversion=off  FilteringAndDerivatives=zero  SimscapeFilterOrder=1  InputFilterTimeConstant=0.001  UdotUserProvided=1
  Six-Pulse Gate Multiplexer : ee_lib/Semiconductors & Converters/Converters/Six-Pulse Gate Multiplexer  port_option=ee.enum.controlport.ps
  g : PMIOPort  Side=Right
  wires:
  Demux/4 -> Simulink-PS Converter4/1
  Demux/3 -> Simulink-PS Converter3/1
  Demux/6 -> Simulink-PS Converter6/1
  Demux/5 -> Simulink-PS Converter5/1
  Demux/2 -> Simulink-PS Converter2/1
  Demux/1 -> Simulink-PS Converter1/1
  s/1 -> Demux/1
  connections:
  Six-Pulse Gate Multiplexer/LConn4 -- Simulink-PS Converter4/RConn1
  Six-Pulse Gate Multiplexer/LConn1 -- Simulink-PS Converter1/RConn1
  Six-Pulse Gate Multiplexer/LConn3 -- Simulink-PS Converter3/RConn1
  Six-Pulse Gate Multiplexer/RConn1 -- g/RConn1
  Simulink-PS Converter6/RConn1 -- Six-Pulse Gate Multiplexer/LConn6
  Six-Pulse Gate Multiplexer/LConn2 -- Simulink-PS Converter2/RConn1
  Six-Pulse Gate Multiplexer/LConn5 -- Simulink-PS Converter5/RConn1

== system MVC2026_sim/Power System - BES & PMSM/Charging system/If Action Subsystem/If Action Subsystem ==
  Action Port : ActionPort  ActionPortLabel=if((u1 > u2(1)) & (u1 < (u2(2))) )
  Constant : Constant  Value=CH.PLUG.IFast
  Iref : Outport
  wires:
  Constant/1 -> Iref/1

== system MVC2026_sim/Power System - BES & PMSM/Charging system/If Action Subsystem/If Action Subsystem3 ==
  Action Port : ActionPort  ActionPortLabel=else
  Constant : Constant  Value=CH.PLUG.ISlow
  Iref : Outport
  wires:
  Constant/1 -> Iref/1

== matlab function MVC2026_sim/Profile generation/Subsystem/MATLAB Function ==
  data: u input; y output; TraceRef parameter
function y = fcn(u, TraceRef)

y = u;

if u<(-TraceRef.PosRef(end)/2)
    y = u + TraceRef.PosRef(end);
elseif u>(TraceRef.PosRef(end)/2)
    y = u - TraceRef.PosRef(end);
end
